simulink model "Tutorial4_model"  (R2021a)
settings: Solver=ode45  StartTime=0.0  StopTime=10  FixedStep=Ts  RelTol=1e-7  EnableMultiTasking=on
libraries: simulink_extras x2
settings Model: Creator=SABA  LastModifiedBy=Manu
settings SolverCC: AlgebraicLoopSolver=TrustRegion
settings DataIOCC: LimitDataPoints=on  SaveFormat=Array  ReturnWorkspaceOutputs=off
settings OptimizationCC: LifeSpan=inf
settings DebuggingCC: SFUnexpectedBacktrackingDiag=warning  SFNoUnconditionalDefaultTransitionDiag=warning  SFExecutionAtInitializationDiag=none  SFMachineParentedDataDiag=warning  ArithmeticOperatorsInVariantConditions=warning
settings HardwareCC: ProdBitPerPointer=32  ProdBitPerSizeT=32  ProdBitPerPtrDiffT=32  ProdLargestAtomicFloat=None  ProdIntDivRoundTo=Undefined  ProdEndianess=Unspecified  ProdWordSize=32  ProdHWDeviceType=32-bit Generic
settings ModelReferenceCC: PropagateSignalLabelsOutOfModel=off
settings SFSimCC: SimUseLocalCustomCode=off  CustomCodeUndefinedFunction=UseInterfaceOnly
settings RTWCC: RTWUseLocalCustomCode=off
settings CodeAppCC: StateflowObjectComments=on
settings GRTTargetCC: TargetLangStandard=C89/C90 (ANSI)
settings ConfigComp: CovMetricSettings=dw  CovSaveCumulativeToWorkspaceVar=on  CovSaveSingleToWorkspaceVar=on  CovExternalEMLEnable=off

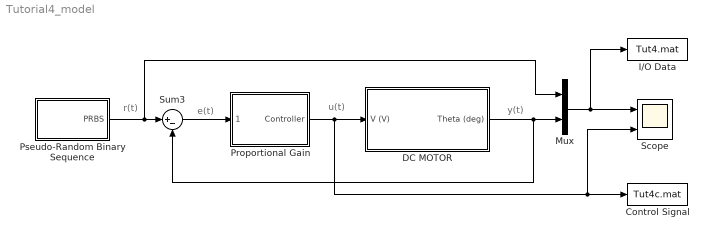
== system Tutorial4_model ==
  note: u(t)
  note: y(t)
  note: r(t)
  note: e(t)
  " DC MOTOR" : Subsystem  TreatAsAtomicUnit=on  mask(DC Servo Motor Module){La=5e-5, Ra=4, Jm=2.5e-7, Bm=1.019e-7, noise=1}
      mask prompts: La "Armature Inductance - La (H)"; Ra "Armature Resistance - Ra (ohm)"; Jm "Motor Inertia - Jm (oz.in.sec^2)"; Bm "Motor Viscous Friction - Bm (N.m.sec)"; noise "Additive Noise (ON = 1, OFF = 0)"
      mask help: The DC Motor model with dead-zone nonlinearities.
      settings: MinAlgLoopOccurrences=on
  Control Signal : ToFile  Filename=Tut4c.mat  MatrixName=cont  SampleTime=1/150
  I/O Data : ToFile  Filename=Tut4.mat  MatrixName=out  SampleTime=1/150
  Mux : Mux  Inputs=2
  Proportional Gain : Subsystem  mask(Controller){Kp=0.75}
      mask prompts: Kp "Proportional Gain (Kp)"
      mask help: Proportional Controller with saturated output. The output limited between -1.4V to +1.4V
      mask DialogControl Parameters Prompt: Parameters
  Pseudo-Random Binary Sequence : Subsystem  mask(DPRBS){N=1500, K=70, A=45}
      mask prompts: N "Number of Sample Points (N)"; K "Switch Constant (K)"; A "Amplitude (A)"
      mask help: Generates a random switching sequence of discrete samples valued at -A and +A.
  Scope : Scope  NumInputPorts=2
  Sum3 : Sum  Inputs=|+-
  wires:
  Pseudo-Random Binary Sequence/1(PRBS) -> Mux/1, Sum3/1
  Mux/1 -> I/O Data/1, Scope/1
  Sum3/1 -> Proportional Gain/1("  ")
  Proportional Gain/1("Controller    ") -> Scope/2, Control Signal/1, " DC MOTOR"/1(V (V))
  " DC MOTOR"/1(Theta (deg)) -> Mux/2, Sum3/2

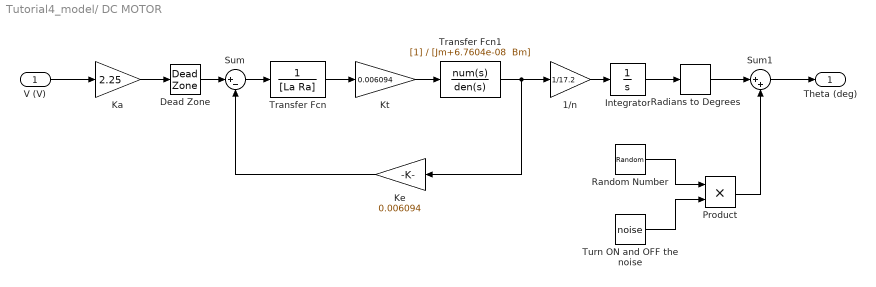
== system Tutorial4_model/ DC MOTOR ==
  V (V) : Inport
  1/n : Gain  Gain=1/17.2
  Dead Zone : DeadZone  LowerValue=-0.026  UpperValue=0.026  ZeroCross=off  SaturateOnIntegerOverflow=on
  Integrator : TransferFcn  Denominator=[1 0]
  Ka : Gain  Gain=2.25
  Ke : Gain  Gain=0.006094
  Kt : Gain  Gain=0.006094
  Product : Product
  Radians to Degrees : simulink_extras/Transformations/Radians to Degrees
  Random Number : RandomNumber  Seed=randi([0 100],1,1)  SampleTime=1/150
  Sum : Sum  Inputs=|+-
  Sum1 : Sum  Inputs=|++
  Transfer Fcn : TransferFcn  Denominator=[La Ra]
  Transfer Fcn1 : TransferFcn  Denominator="[Jm+6.7604e-08  Bm]"
  Turn ON and OFF the noise : Constant  Value=noise  SampleTime=1/150
  Theta (deg) : Outport
  wires:
  Sum/1 -> Transfer Fcn/1
  Integrator/1 -> Radians to Degrees/1
  Transfer Fcn/1 -> Kt/1
  Kt/1 -> Transfer Fcn1/1
  Transfer Fcn1/1 -> Ke/1, 1/n/1
  1/n/1 -> Integrator/1
  Ke/1 -> Sum/2
  Ka/1 -> Dead Zone/1
  V (V)/1 -> Ka/1
  Dead Zone/1 -> Sum/1
  Radians to Degrees/1 -> Sum1/1
  Sum1/1 -> Theta (deg)/1
  Random Number/1 -> Product/1
  Turn ON and OFF the noise/1 -> Product/2
  Product/1 -> Sum1/2

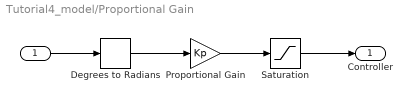
== system Tutorial4_model/Proportional Gain ==
  "  " : Inport
  Degrees to Radians : simulink_extras/Transformations/Degrees to Radians
  Proportional Gain : Gain  Gain=Kp
  Saturation : Saturate  UpperLimit=1.4  LowerLimit=-1.4  ZeroCross=off
  "Controller    " : Outport
  wires:
  "  "/1 -> Degrees to Radians/1
  Proportional Gain/1 -> Saturation/1
  Degrees to Radians/1 -> Proportional Gain/1
  Saturation/1 -> "Controller    "/1

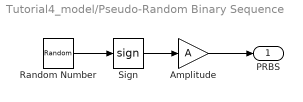
== system Tutorial4_model/Pseudo-Random Binary Sequence ==
  Amplitude : Gain  Gain=A
  Random Number : RandomNumber  Seed=randi([0 100],1,1)  SampleTime=10*K/N
  Sign : Signum
  PRBS : Outport
  wires:
  Sign/1 -> Amplitude/1
  Random Number/1 -> Sign/1
  Amplitude/1 -> PRBS/1
